simulink model "Task1"  (R2022a)
settings: Solver=FixedStepAuto  StartTime=0.0  StopTime=20  FixedStep=0.0001  RelTol=1e-3
undefined symbols (not defined in the file): wcoeff, wucoeff
settings Model: Creator=Family  LastModifiedBy=Family

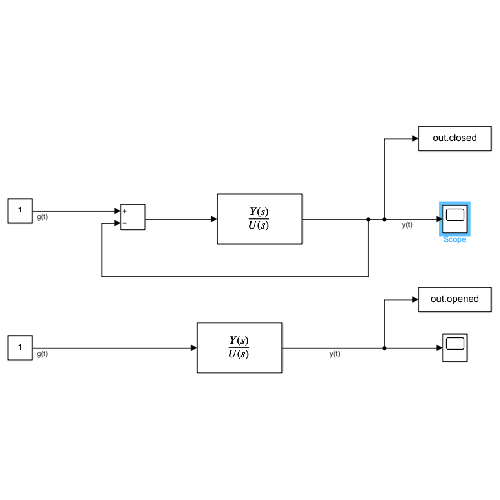
[thumbnail: Simulink's stored preview of the top-level diagram]
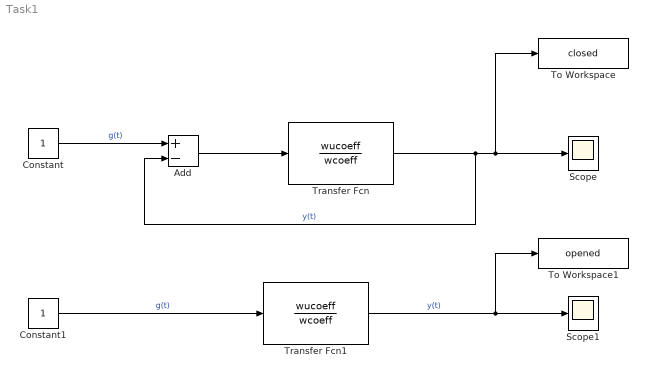
== system Task1 ==
  Add : Sum  Inputs=+-
  Constant : Constant  SampleTime=-1
  Constant1 : Constant  SampleTime=-1
  Scope : Scope
  Scope1 : Scope
  To Workspace : ToWorkspace  VariableName=closed  SaveFormat=Timeseries  SampleTime=-1
  To Workspace1 : ToWorkspace  VariableName=opened  SaveFormat=Timeseries  SampleTime=-1
  Transfer Fcn : TransferFcn  Numerator=wucoeff  Denominator=wcoeff
  Transfer Fcn1 : TransferFcn  Numerator=wucoeff  Denominator=wcoeff
  wires:
  Transfer Fcn/1 -> Add/2, To Workspace/1, Scope/1  "y(t)"
  Constant/1 -> Add/1  "g(t)"
  Add/1 -> Transfer Fcn/1
  Constant1/1 -> Transfer Fcn1/1  "g(t)"
  Transfer Fcn1/1 -> To Workspace1/1, Scope1/1  "y(t)"
